simulink model "GridConnectInverterController"  (R2020a)
settings: Solver=VariableStepAuto  StartTime=0.0  StopTime=10.0  RelTol=1e-3
settings Model: DataDictionary=PCS_Simulation_EnviromentDD.sldd  Creator=ykamatan  LastModifiedBy=ykamatan

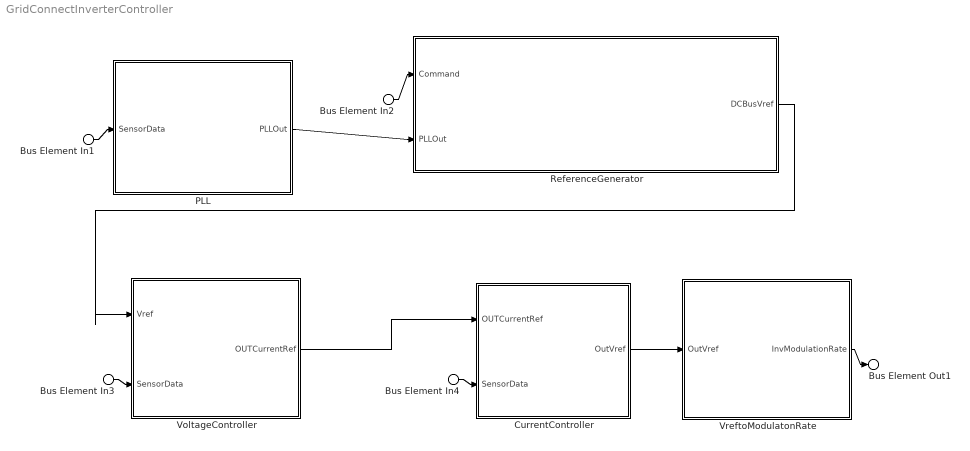
== system GridConnectInverterController ==
  Bus Element In2 : Inport  PortName=Command
  Bus Element In1 : Inport  Port=2  PortName=SensorData  Element=PVOutVoltage
  Bus Element In3 : Inport  Port=2  PortName=SensorData  Element=DCBusVoltage
  Bus Element In4 : Inport  Port=2  PortName=SensorData  Element=InvOutCurrent
  CurrentController : Subsystem
      settings: PortSchema="{\"entries\":[{\"content\":{\"headerSize\":26,\"margin\":15,\"minimumSpacing\":25,\"sides\":[{\"content\":{\"connectorIds\":[\"In1\",\"In2\"]},\"type\":\"ConnectorPlacement.EquallySpacedRectSide\",\"uuid\":\"4a276d0d-1e61-4fe0-a236-83af253ddea3\"},{\"content\":{\"connectorIds\":[\"Out1\"],\"side\":\"RIGHT\"},\"type\":\"ConnectorPlacement.EquallySpacedRectSide\",\"uuid\":\"2cace6bb-f607-4cf0-88cb-c27cbcb348d0\"},{\"content\":{\"connectorIds\":[],\"side\":\"TOP\"},\"type\":\"ConnectorPlacement.EquallySpacedRectSide\",\"uuid\":\"e006ff0e-17df-4e20-869a-e198fc913bc1\"}]},\"type\":\"ConnectorPlacement.EquallySpacedConnector\",\"uuid\":\"089f71ad-781e-4fba-9ec7-6f61de1efbd5\"}],\"packageUris\":[\"http://schema.mathworks.com/mf0/Connector/19700101\"],\"version\":\"1.0\"}"
  PLL : Subsystem
      settings: PortSchema="{\"entries\":[{\"content\":{\"headerSize\":26,\"margin\":15,\"minimumSpacing\":25,\"sides\":[{\"content\":{\"connectorIds\":[\"In1\"]},\"type\":\"ConnectorPlacement.EquallySpacedRectSide\",\"uuid\":\"4a276d0d-1e61-4fe0-a236-83af253ddea3\"},{\"content\":{\"connectorIds\":[\"Out1\"],\"side\":\"RIGHT\"},\"type\":\"ConnectorPlacement.EquallySpacedRectSide\",\"uuid\":\"2cace6bb-f607-4cf0-88cb-c27cbcb348d0\"},{\"content\":{\"connectorIds\":[],\"side\":\"TOP\"},\"type\":\"ConnectorPlacement.EquallySpacedRectSide\",\"uuid\":\"e006ff0e-17df-4e20-869a-e198fc913bc1\"}]},\"type\":\"ConnectorPlacement.EquallySpacedConnector\",\"uuid\":\"089f71ad-781e-4fba-9ec7-6f61de1efbd5\"}],\"packageUris\":[\"http://schema.mathworks.com/mf0/Connector/19700101\"],\"version\":\"1.0\"}"
  ReferenceGenerator : Subsystem
      settings: PortSchema="{\"entries\":[{\"content\":{\"headerSize\":26,\"margin\":15,\"minimumSpacing\":25,\"sides\":[{\"content\":{\"connectorIds\":[\"In1\",\"In2\"]},\"type\":\"ConnectorPlacement.EquallySpacedRectSide\",\"uuid\":\"4a276d0d-1e61-4fe0-a236-83af253ddea3\"},{\"content\":{\"connectorIds\":[\"Out1\"],\"side\":\"RIGHT\"},\"type\":\"ConnectorPlacement.EquallySpacedRectSide\",\"uuid\":\"2cace6bb-f607-4cf0-88cb-c27cbcb348d0\"},{\"content\":{\"connectorIds\":[],\"side\":\"TOP\"},\"type\":\"ConnectorPlacement.EquallySpacedRectSide\",\"uuid\":\"e006ff0e-17df-4e20-869a-e198fc913bc1\"},{\"content\":{\"connectorIds\":[],\"side\":\"BOTTOM\"},\"type\":\"ConnectorPlacement.EquallySpacedRectSide\",\"uuid\":\"b60a2369-74d8-4221-8534-b8b37938a883\"}]},\"type\":\"ConnectorPlacement.EquallySpacedConnector\",\"uuid\":\"089f71ad-781e-4fba-9ec7-6f61de1efbd5\"}],\"packageUris\":[\"http://schema.mathworks.com/mf0/Connector/19700101\"],\"version\":\"1.0\"}"
  VoltageController : Subsystem
      settings: PortSchema="{\"entries\":[{\"content\":{\"headerSize\":26,\"margin\":15,\"minimumSpacing\":25,\"sides\":[{\"content\":{\"connectorIds\":[\"In1\",\"In2\"]},\"type\":\"ConnectorPlacement.EquallySpacedRectSide\",\"uuid\":\"4a276d0d-1e61-4fe0-a236-83af253ddea3\"},{\"content\":{\"connectorIds\":[\"Out1\"],\"side\":\"RIGHT\"},\"type\":\"ConnectorPlacement.EquallySpacedRectSide\",\"uuid\":\"2cace6bb-f607-4cf0-88cb-c27cbcb348d0\"},{\"content\":{\"connectorIds\":[],\"side\":\"TOP\"},\"type\":\"ConnectorPlacement.EquallySpacedRectSide\",\"uuid\":\"e006ff0e-17df-4e20-869a-e198fc913bc1\"}]},\"type\":\"ConnectorPlacement.EquallySpacedConnector\",\"uuid\":\"089f71ad-781e-4fba-9ec7-6f61de1efbd5\"}],\"packageUris\":[\"http://schema.mathworks.com/mf0/Connector/19700101\"],\"version\":\"1.0\"}"
  VreftoModulatonRate : Subsystem
      settings: PortSchema="{\"entries\":[{\"content\":{\"headerSize\":26,\"margin\":15,\"minimumSpacing\":25,\"sides\":[{\"content\":{\"connectorIds\":[\"In1\"]},\"type\":\"ConnectorPlacement.EquallySpacedRectSide\",\"uuid\":\"4a276d0d-1e61-4fe0-a236-83af253ddea3\"},{\"content\":{\"connectorIds\":[\"Out1\"],\"side\":\"RIGHT\"},\"type\":\"ConnectorPlacement.EquallySpacedRectSide\",\"uuid\":\"2cace6bb-f607-4cf0-88cb-c27cbcb348d0\"},{\"content\":{\"connectorIds\":[],\"side\":\"TOP\"},\"type\":\"ConnectorPlacement.EquallySpacedRectSide\",\"uuid\":\"e006ff0e-17df-4e20-869a-e198fc913bc1\"}]},\"type\":\"ConnectorPlacement.EquallySpacedConnector\",\"uuid\":\"089f71ad-781e-4fba-9ec7-6f61de1efbd5\"}],\"packageUris\":[\"http://schema.mathworks.com/mf0/Connector/19700101\"],\"version\":\"1.0\"}"
  Bus Element Out1 : Outport  PortName=InvModulationRate
  wires:
  Bus Element In1/1 -> PLL/1(SensorData)
  Bus Element In3/1 -> VoltageController/2(SensorData)
  ReferenceGenerator/1(DCBusVref) -> VoltageController/1(Vref)
  Bus Element In4/1 -> CurrentController/2(SensorData)
  VoltageController/1(OUTCurrentRef) -> CurrentController/1(OUTCurrentRef)
  PLL/1(PLLOut) -> ReferenceGenerator/2(PLLOut)
  CurrentController/1(OutVref) -> VreftoModulatonRate/1(OutVref)
  VreftoModulatonRate/1(InvModulationRate) -> Bus Element Out1/1
  Bus Element In2/1 -> ReferenceGenerator/1(Command)

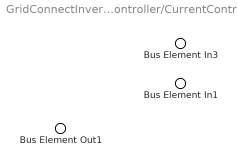
== system GridConnectInverterController/CurrentController ==
  Bus Element In3 : Inport  PortName=OUTCurrentRef
  Bus Element In1 : Inport  Port=2  PortName=SensorData
  Bus Element Out1 : Outport  PortName=OutVref

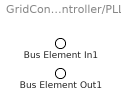
== system GridConnectInverterController/PLL ==
  Bus Element In1 : Inport  PortName=SensorData
  Bus Element Out1 : Outport  PortName=PLLOut

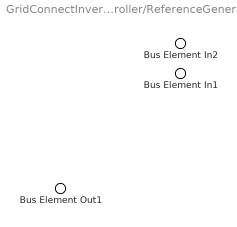
== system GridConnectInverterController/ReferenceGenerator ==
  Bus Element In1 : Inport  PortName=Command
  Bus Element In2 : Inport  Port=2  PortName=PLLOut
  Bus Element Out1 : Outport  PortName=DCBusVref

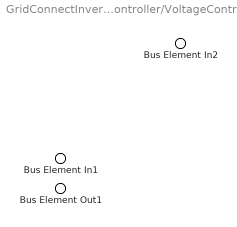
== system GridConnectInverterController/VoltageController ==
  Bus Element In2 : Inport  PortName=Vref
  Bus Element In1 : Inport  Port=2  PortName=SensorData
  Bus Element Out1 : Outport  PortName=OUTCurrentRef

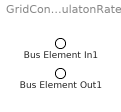
== system GridConnectInverterController/VreftoModulatonRate ==
  Bus Element In1 : Inport  PortName=OutVref
  Bus Element Out1 : Outport  PortName=InvModulationRate
